simulink model "FormationSImulation6"  (R2024a)
settings: Solver=VariableStepAuto  StartTime=0.0  StopTime=60*60*2  RelTol=1e-3
libraries: nesl_utility x8, fl_lib x7
settings Model: Creator=DELL  LastModifiedBy=DELL

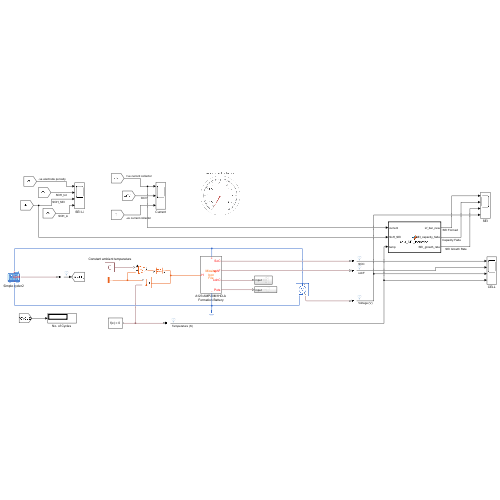
[thumbnail: Simulink's stored preview of the top-level diagram]
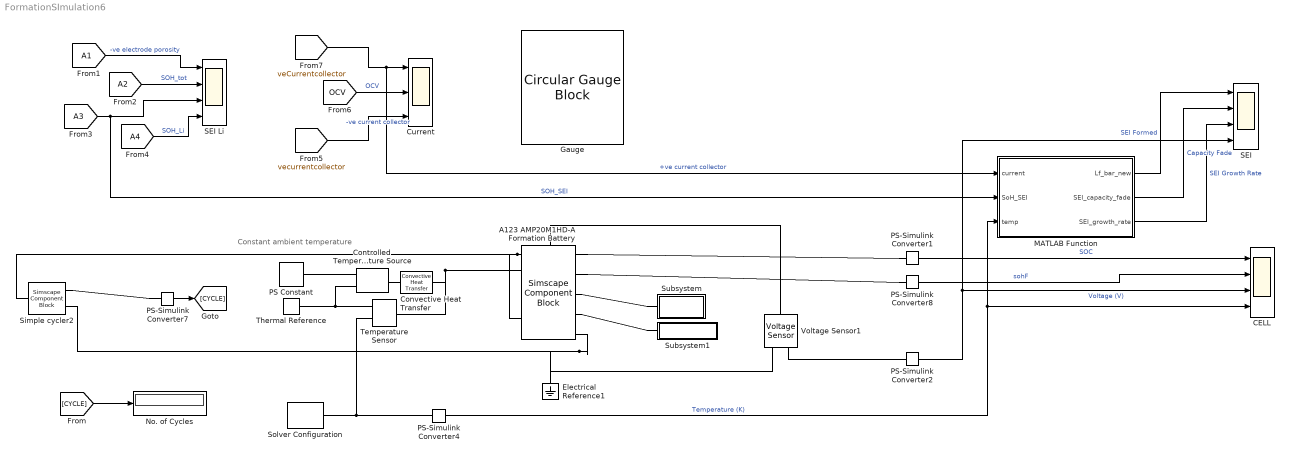
== system FormationSImulation6 ==
  note: Constant ambient temperature
  A123 AMP20M1HD-A Formation Battery : SimscapeComponentBlock  SourceFile=OriginalTSPMeA_A123  ComponentPath=OriginalTSPMeA_A123  ComponentVariants="[\"OriginalTSPMeA_A123\"]"  ComponentVariantNames="[\"OriginalTSPMeA_A123\"]"  ClassName=OriginalTSPMeA_A123  SchemaVersion=1  z0=0.05  T0=298 K  eps_n0=0.25  Lf0=1 um  Cn=19.6 A*hr  DnRef=3.3E-14 m^2/s  DpRef=4E-15 m^2/s  sigma_nRef=215 S/m  sigma_eRef=1.2 S/m  sigma_pRef=0.18 S/m  tr=0.2594  ce0=1000 mol/m^3  cn_max=33133 mol/m^3  cp_max=63104 mol/m^3  sn_max=0.9014  sn_min=0.0279  sp_max=0.9072  sp_min=0.2567  knRef=6.48E-7 A*m^(5/2)/mol^(3/2)  kpRef=3.42E-6 A*m^(5/2)/mol^(3/2)  Cp=110 J/K  Tref=298 K  Ea_kn=1 kJ/mol  Ea_kp=1 kJ/mol  Ea_Dn=75 kJ/mol  Ea_De=1.2 kJ/mol  Ea_Dp=10 kJ/mol  Ea_sigman=80 kJ/mol  Ea_sigmae=80 kJ/mol  Ea_sigmap=80 kJ/mol  Ea_ksei=1 kJ/mol  Ea_Dsei=1 kJ/mol  Ea_sigmasei=1 kJ/mol  Ea_kLi=1 kJ/mol  kseiRef=1E-11 m/s  DseiRef=2E-19 m^2/s  sigma_seiRef=5E-6 S/m  Msei=0.162 kg/mol  pho_sei=1690 kg/m^3  Usei=1 V  csei0=1 mol/m^3  kLiRef=1E-11 m/s  ULi=0 V  MLi=6.94E-3 kg/mol  pho_Li=534 kg/m^3  Ln=85.2 um  Ls=12 um  Lp=75.6 um  Area_p=1027 cm^2  eps_s=0.47  eps_p=0.335  Rn=5.86 um  Rp=5.22 um  an=3.84E5 1/m  ap=3.82E5 1/m
      settings: CopyFcn=simscape.engine.sli.internal.componentblockcallback(gcbh,'COPY')  PreCopyFcn=simscape.engine.sli.internal.componentblockcallback(gcbh,'PRECOPY')  PreDeleteFcn=simscape.engine.sli.internal.componentblockcallback(gcbh,'PREDELETE')  InternalSimscapePortConfiguration="{\"Bottom\":[{\"id\":\"n\",\"label\":\"-\",\"type\":\"foundation.electrical.electrical\"}],\"Left\":[{\"id\":\"Hi\",\"label\":\"H\",\"type\":\"foundation.thermal.thermal\"}],\"Right\":[{\"id\":\"z\",\"label\":\"SoC\",\"type\":\"output\"},{\"id\":\"Lf_bar\",\"label\":\"sohF\",\"type\":\"output\"},{\"id\":\"SoH_Cn\",\"label\":\"sohC\",\"type\":\"output\"},{\"id\":\"pots\",\"label\":\"Pots\",\"type\":\"output\"}],\"Top\":[{\"id\":\"p\",\"label\":\"+\",\"type\":\"foundation.electrical.electrical\"}]}"
      mask Type: TSPMeA
  CELL : Scope  NumInputPorts=4
  Controlled Temperature Source : fl_lib/Thermal/Thermal Sources/Controlled Temperature Source
  Convective Heat Transfer : fl_lib/Thermal/Thermal Elements/Convective Heat Transfer  thermal_type=foundation.enum.constant_variable.constant  area=0.064 m^2  heat_tr_coeff=5 W/(K*m^2)  min_heat_tr_coeff=1e-3 W/(K*m^2)  T_specify=off  T_priority=None  T=0 K  T_nominal_specify=off  T_nominal_value=1  T_nominal_unit=K  Q_specify=off  Q_priority=None  Q=0 W  Q_nominal_specify=off  Q_nominal_value=1  Q_nominal_unit=W
  Current : Scope  NumInputPorts=3
  Electrical Reference1 : fl_lib/Electrical/Electrical Elements/Electrical Reference
  Gauge : CircularGaugeBlock  ScaleMax=5
  MATLAB Function : MATLAB Function  TreatAsAtomicUnit=on
  "No. of Cycles " : Display
  PS Constant : fl_lib/Physical Signals/Sources/PS Constant  constant=298 K
  PS-Simulink Converter{1..2,4,7..8} (5 alike) : nesl_utility/PS-Simulink Converter  PhysicalDomain=network_engine_domain  SubClassName=ps_output  LeftPortType=input  RightPortType=output  PseudoPeriodic=off  Frequencies=[]  VectorFormat=inherit  Unit=inherit  AffineConversion=off
  SEI : Scope  NumInputPorts=4
  SEI Li : Scope  NumInputPorts=4
  Simple cycler2 : SimscapeComponentBlock  SourceFile=BatteryLibrary.Utilities.BatteryCycler  ComponentPath=BatteryLibrary.Utilities.BatteryCycler  ComponentVariants="[\"BatteryLibrary.Utilities.BatteryCycler\"]"  ComponentVariantNames="[\"BatteryCycler\"]"  ClassName=BatteryCycler  SchemaVersion=1  Vmax=3.6 V  Vmin=2.0 V  Ic=0.2 A  Ico=0.05 A  Id=-6 A  tRestC=1800 s  tRestD=1800 s
      settings: CopyFcn=simscape.engine.sli.internal.componentblockcallback(gcbh,'COPY')  PreCopyFcn=simscape.engine.sli.internal.componentblockcallback(gcbh,'PRECOPY')  PreDeleteFcn=simscape.engine.sli.internal.componentblockcallback(gcbh,'PREDELETE')  InternalSimscapePortConfiguration="{\"Bottom\":[{\"id\":\"n\",\"label\":\"-\",\"type\":\"foundation.electrical.electrical\"}],\"Left\":[],\"Right\":[{\"id\":\"numCyc\",\"label\":\"Cyc#\",\"type\":\"output\"}],\"Top\":[{\"id\":\"p\",\"label\":\"+\",\"type\":\"foundation.electrical.electrical\"}]}"
      mask Type: A simple battery cycler
  Solver Configuration : nesl_utility/Solver Configuration  PhysicalDomain=network_engine_domain  SubClassName=solver  LeftPortType=input  RightPortType=generic  Tones=[]  Harmonics=[]  SimulateNoise=off  Profile=off  UseLocalSampling=off  EnableSwitchedLinearOptims=on  FrequencyDomain=off  UseCCode=off  RelTol=0.001  AbsTol=0.001  MinStep=1e-09  ToWorkspace=off  RevertToSquareIcSolve=off  NumHomotopyIterations=100  PhasorMode=off  PhasorModeNumHarmonics=1  ConsistencySolver=NEWTON_XTOL_AFTER_FTOL  IndexReductionMethod=DerivativeReplacement  DoDC=off  ResidualTolerance=1e-09  ConsistencyTolSource=GLOBAL  ConsistencyAbsTol=0.001  ConsistencyRelTol=0.001  ConsistencyTolFactor=0.001  UseLocalSolver=on  LocalSolverChoice=NE_BACKWARD_EULER_ADVANCER  ResolveIndetEquations=on  FunctionEvalNumThread=1  LocalSolverSampleTime=1  DoFixedCost=on  MaxNonlinIter=3  MaxModeIter=2  ComputeImpulses=off  ImpulseIterations=2  LinearAlgebra=auto  LinearAlgebraNumThread=0  EquationFormulation=NE_TIME_EF  DelaysMemoryBudget=1024  AutomaticFiltering=on  FilteringTimeConstant=0.001  PartitionStorageMethod=AS_NEEDED  PartitionMemoryBudget=1024  PartitionMethod=ROBUST  MultibodyUseLocalSolver=off  MultibodyLocalSolverChoice=ODE1  MultibodyLocalSolverSampleTime=0.001
  Subsystem : Subsystem
  Subsystem1 : Subsystem
  Temperature Sensor : fl_lib/Thermal/Thermal Sensors/Temperature Sensor  temperature_measure=foundation.enum.MeasurementReference.difference
  Thermal Reference : fl_lib/Thermal/Thermal Elements/Thermal Reference
  Voltage Sensor1 : fl_lib/Electrical/Electrical Sensors/Voltage Sensor
  wires:
  [vecurrentcollector] -> Current/3  "-ve current collector"
  [CYCLE] -> "No. of Cycles "/1
  [A4] -> SEI Li/4  "SOH_Li"
  [A1] -> SEI Li/1  "-ve electrode porosity"
  [OCV] -> Current/2  "OCV"
  PS-Simulink Converter4/1 -> CELL/4, MATLAB Function/3(temp)  "Temperature (K)"
  PS-Simulink Converter7/1 -> [CYCLE]
  [veCurrentcollector] -> MATLAB Function/1(current), Current/1  "+ve current collector"
  [A2] -> SEI Li/2  "SOH_tot"
  [A3] -> MATLAB Function/2(SoH_SEI), SEI Li/3  "SOH_SEI"
  MATLAB Function/1(Lf_bar_new) -> SEI/1  "SEI Formed"
  MATLAB Function/2(SEI_capacity_fade) -> SEI/2  "Capacity Fade"
  MATLAB Function/3(SEI_growth_rate) -> SEI/3  "SEI Growth Rate"
  PS-Simulink Converter2/1 -> CELL/3, SEI/4  "Voltage (V)"
  PS-Simulink Converter1/1 -> CELL/1  "SOC"
  PS-Simulink Converter8/1 -> CELL/2  "sohF"
  connections:
  Simple cycler2/RConn2 -- Voltage Sensor1/RConn2 -- A123 AMP20M1HD-A Formation Battery/RConn5 -- Electrical Reference1/LConn1
  Simple cycler2/LConn1 -- Voltage Sensor1/LConn1 -- A123 AMP20M1HD-A Formation Battery/LConn2
  Solver Configuration/RConn1 -- Temperature Sensor/RConn2 -- PS-Simulink Converter4/LConn1
  A123 AMP20M1HD-A Formation Battery/LConn1 -- Temperature Sensor/LConn1 -- Convective Heat Transfer/LConn1
  Voltage Sensor1/RConn1 -- PS-Simulink Converter2/LConn1
  Controlled Temperature Source/RConn2 -- Temperature Sensor/RConn1 -- Thermal Reference/LConn1
  Subsystem1/LConn1 -- A123 AMP20M1HD-A Formation Battery/RConn4
  Subsystem/LConn1 -- A123 AMP20M1HD-A Formation Battery/RConn3
  A123 AMP20M1HD-A Formation Battery/RConn1 -- PS-Simulink Converter1/LConn1
  PS Constant/RConn1 -- Controlled Temperature Source/RConn1
  A123 AMP20M1HD-A Formation Battery/RConn2 -- PS-Simulink Converter8/LConn1
  PS-Simulink Converter7/LConn1 -- Simple cycler2/RConn1
  Controlled Temperature Source/LConn1 -- Convective Heat Transfer/RConn1

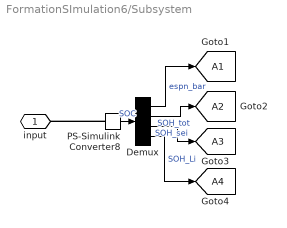
== system FormationSImulation6/Subsystem ==
  Demux : Demux
  PS-Simulink Converter8 : nesl_utility/PS-Simulink Converter  PhysicalDomain=network_engine_domain  SubClassName=ps_output  LeftPortType=input  RightPortType=output  PseudoPeriodic=off  Frequencies=[]  VectorFormat=inherit  Unit=inherit  AffineConversion=off
  input : PMIOPort  Side=Left
  tag scope: A1=global, A2=global, A3=global, A4=global
  wires:
  PS-Simulink Converter8/1 -> Demux/1  "SOC"
  Demux/2 -> [A2]  "SOH_tot"
  Demux/1 -> [A1]  "espn_bar"
  Demux/3 -> [A3]  "SOH_sei"
  Demux/4 -> [A4]  "SOH_Li"
  connections:
  PS-Simulink Converter8/LConn1 -- input/RConn1

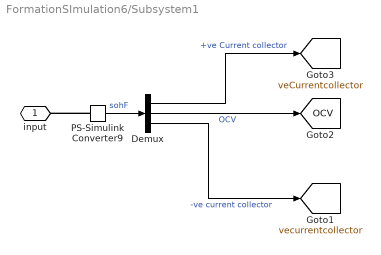
== system FormationSImulation6/Subsystem1 ==
  Demux : Demux  Outputs=3
  PS-Simulink Converter9 : nesl_utility/PS-Simulink Converter  PhysicalDomain=network_engine_domain  SubClassName=ps_output  LeftPortType=input  RightPortType=output  PseudoPeriodic=off  Frequencies=[]  VectorFormat=inherit  Unit=inherit  AffineConversion=off
  input : PMIOPort  Side=Left
  tag scope: OCV=global, veCurrentcollector=global, vecurrentcollector=global
  wires:
  PS-Simulink Converter9/1 -> Demux/1  "sohF"
  Demux/2 -> [OCV]  "OCV"
  Demux/1 -> [veCurrentcollector]  "+ve Current collector"
  Demux/3 -> [vecurrentcollector]  "-ve current collector"
  connections:
  PS-Simulink Converter9/LConn1 -- input/RConn1

== matlab function FormationSImulation6/MATLAB Function ==
  data: current input; Lf_bar_new output; SoH_SEI input; temp input; SEI_capacity_fade output; SEI_growth_rate output
function [Lf_bar_new, SEI_capacity_fade, SEI_growth_rate] = calc_SEI_formation(current, SoH_SEI, temp)
    % Constants
    %F = 96485;           % Faraday constant [C/mol]
    R = 8.314;           % Universal gas constant [J/K/mol]
    time_step = 10;         % Time step for SEI growth [s]
    k_SEI = 1e-6;           % SEI growth rate constant [m/s]
    %A = 0.1;                % Electrode surface area [m^2]
    E_a = 50000;            % Activation energy for SEI formation [J/mol]

    
    % SEI growth rate equation: dLf/dt = k_SEI * I * exp(-Ea/(R*T))
    SEI_growth_rate = k_SEI * abs(current) * exp(-E_a / (R * temp)); % [m/s]
    
    % Update SEI film thickness over time
    Lf_bar_new = SoH_SEI + SEI_growth_rate * time_step; % SEI thickness [m]
    
    % Calculate SEI contribution to capacity fade (assuming proportional relation)
    SEI_contrib = SEI_growth_rate * time_step; % SEI contribution to capacity fade
    
    % Update total capacity fade due to SEI formation
    SEI_capacity_fade = SoH_SEI + SEI_contrib;
   
end
